simulink model "dcmotor_g11_compare"  (R2025b)
settings: Solver=VariableStepAuto  StartTime=0.0  StopTime=10.0  RelTol=1e-3
values from neighbouring files (symbols this model uses):
  A = [0 1 0 ... (first row only)    [dc_motor_g11_ss_tf_canonical.m]
  Atilde = [0 1 ... (first row only)    [dc_motor_g11_ss_tf_canonical.m]
  B = [0 0 ... (first row only)    [dc_motor_g11_ss_tf_canonical.m]
  Btilde = [0 ... (first row only)    [dc_motor_g11_ss_tf_canonical.m]
  C = [0 1 0 ... (first row only)    [dc_motor_g11_ss_tf_canonical.m]
  Ctilde = [b0 b1]    [dc_motor_g11_ss_tf_canonical.m]
  D = zeros(3,2)    [dc_motor_g11_ss_tf_canonical.m]
  Dtilde = [0]    [dc_motor_g11_ss_tf_canonical.m]
  GV_den = [Jm*La c*La+Jm*R+Jm*Rm KT*KV+c*R+c*Rm]    [dc_motor_g11_ss_tf_canonical.m]
  GV_num = [KT]    [dc_motor_g11_ss_tf_canonical.m]
undefined symbols (not defined in the file or in its folder): Atilde2, Btilde2, Ctilde2, Dtilde2
settings Model: Creator=nuris  LastModifiedBy=nuris

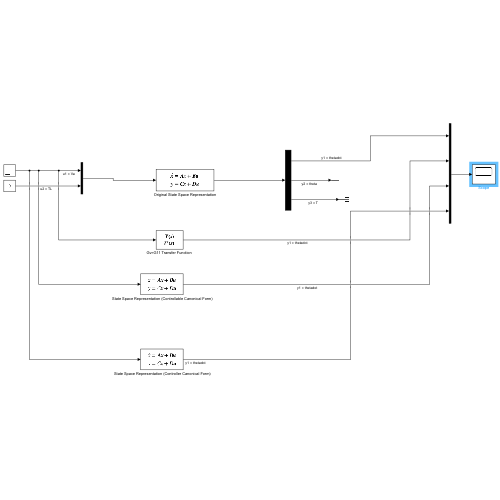
[thumbnail: Simulink's stored preview of the top-level diagram]
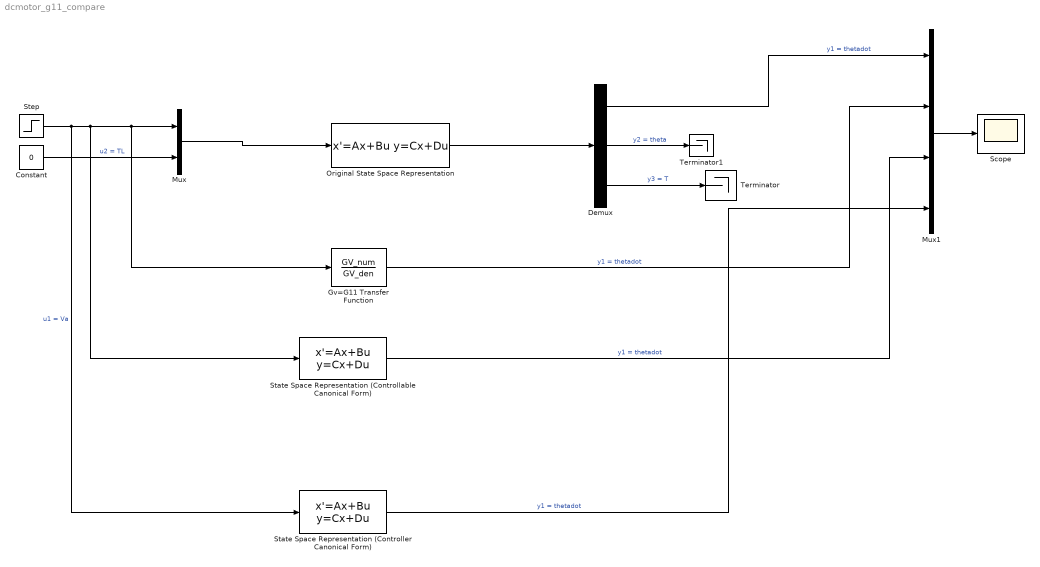
== system dcmotor_g11_compare ==
  " State Space Representation (Controllable Canonical Form)" : StateSpace  A=Atilde  B=Btilde  C=Ctilde  D=Dtilde  InitialCondition=0
  " State Space Representation (Controller Canonical Form)" : StateSpace  A=Atilde2  B=Btilde2  C=Ctilde2  D=Dtilde2  InitialCondition=0
  Constant : Constant  Value=0
  Demux : Demux  Outputs=3
  "Gv=G11 Transfer Function " : TransferFcn  Numerator=GV_num  Denominator=GV_den
  Mux : Mux  Inputs=2
  Mux1 : Mux
  Original State Space Representation : StateSpace  A=A  B=B  C=C  D=D  InitialCondition=0
  Scope : Scope
      settings: ActiveDisplayYMinimum=-2.3162959051863021  ActiveDisplayYMaximum=11.416938696210167
  Step : Step  SampleTime=0
  Terminator : Terminator
  Terminator1 : Terminator
  wires:
  Original State Space Representation/1 -> Demux/1
  Demux/1 -> Mux1/1  "y1 = thetadot"
  Demux/2 -> Terminator1/1  "y2 = theta"
  Demux/3 -> Terminator/1  "y3 = T"
  Step/1 -> " State Space Representation (Controller Canonical Form)"/1, " State Space Representation (Controllable Canonical Form)"/1, "Gv=G11 Transfer Function "/1, Mux/1  "u1 = Va"
  Constant/1 -> Mux/2  "u2 = TL"
  Mux/1 -> Original State Space Representation/1
  "Gv=G11 Transfer Function "/1 -> Mux1/2  "y1 = thetadot"
  Mux1/1 -> Scope/1
  " State Space Representation (Controllable Canonical Form)"/1 -> Mux1/3  "y1 = thetadot"
  " State Space Representation (Controller Canonical Form)"/1 -> Mux1/4  "y1 = thetadot"
